simulink model "Proyecto_LazoAbierto"  (R2024b)
settings: Solver=VariableStepAuto  StartTime=0.0  StopTime=10.0  RelTol=1e-3
settings Model: Creator=Dario  LastModifiedBy=Dario

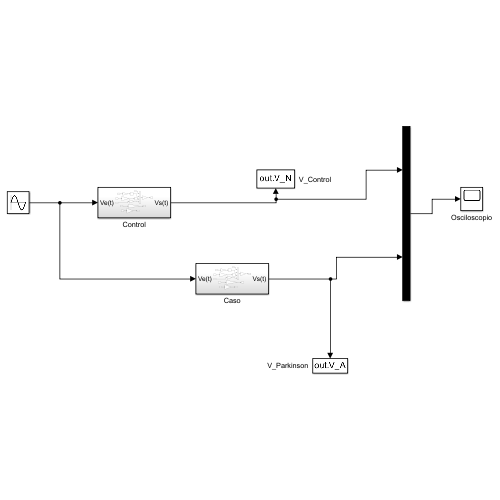
[thumbnail: Simulink's stored preview of the top-level diagram]
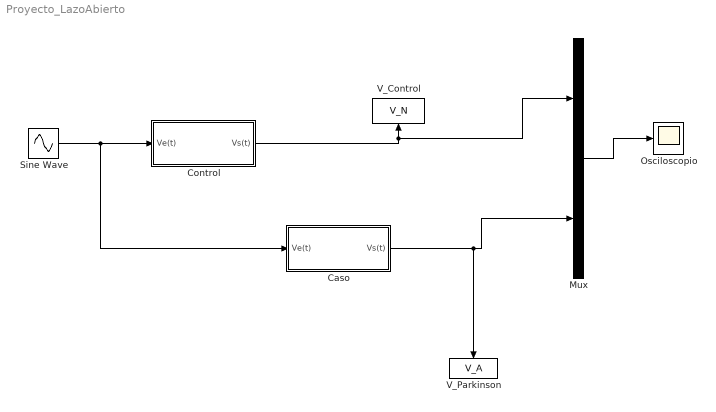
== system Proyecto_LazoAbierto ==
  Caso : Subsystem
  Control : Subsystem
  Mux : Mux  Inputs=2
  Osciloscopio : Scope
  Sine Wave : Sin  Amplitude=5  Frequency=4  SampleTime=0
  V_Control : ToWorkspace  VariableName=V_N  SampleTime=-1
  V_Parkinson : ToWorkspace  VariableName=V_A  SampleTime=-1
  wires:
  Sine Wave/1 -> Caso/1(Ve(t)), Control/1(Ve(t))
  Control/1(Vs(t)) -> Mux/1, V_Control/1
  Mux/1 -> Osciloscopio/1
  Caso/1(Vs(t)) -> V_Parkinson/1, Mux/2

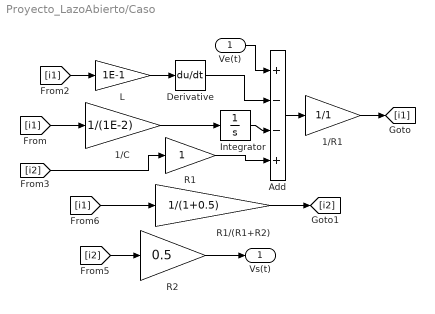
== system Proyecto_LazoAbierto/Caso ==
  Ve(t) : Inport
  1/C : Gain  Gain=1/(1E-2)
  1/R1 : Gain  Gain=1/1
  Add : Sum  Inputs=+--+
  Derivative : Derivative
  Integrator : Integrator
  L : Gain  Gain=1E-1
  R1 : Gain
  R1/(R1+R2) : Gain  Gain=1/(1+0.5)
  R2 : Gain  Gain=0.5
  Vs(t) : Outport
  wires:
  [i1] -> L/1
  Derivative/1 -> Add/2
  Add/1 -> 1/R1/1
  1/C/1 -> Integrator/1
  R1/(R1+R2)/1 -> [i2]
  [i2] -> R2/1
  R2/1 -> Vs(t)/1
  1/R1/1 -> [i1]
  Ve(t)/1 -> Add/1
  Integrator/1 -> Add/3
  R1/1 -> Add/4
  [i2] -> R1/1
  [i1] -> 1/C/1
  L/1 -> Derivative/1
  [i1] -> R1/(R1+R2)/1

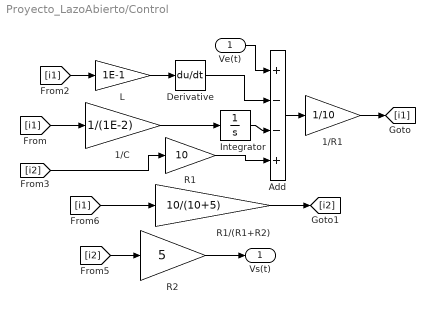
== system Proyecto_LazoAbierto/Control ==
  Ve(t) : Inport
  1/C : Gain  Gain=1/(1E-2)
  1/R1 : Gain  Gain=1/10
  Add : Sum  Inputs=+--+
  Derivative : Derivative
  Integrator : Integrator
  L : Gain  Gain=1E-1
  R1 : Gain  Gain=10
  R1/(R1+R2) : Gain  Gain=10/(10+5)
  R2 : Gain  Gain=5
  Vs(t) : Outport
  wires:
  Integrator/1 -> Add/3
  [i2] -> R2/1
  R2/1 -> Vs(t)/1
  1/R1/1 -> [i1]
  Ve(t)/1 -> Add/1
  [i1] -> 1/C/1
  [i2] -> R1/1
  [i1] -> R1/(R1+R2)/1
  R1/1 -> Add/4
  L/1 -> Derivative/1
  1/C/1 -> Integrator/1
  Derivative/1 -> Add/2
  [i1] -> L/1
  Add/1 -> 1/R1/1
  R1/(R1+R2)/1 -> [i2]
